simulink model "dynamic_mask_example"  (R2013a)
settings: Solver=VariableStepDiscrete  StartTime=0.0  StopTime=10.0  RelTol=1e-3
settings Model: Creator=bbhattac  LastModifiedBy=bbhattac

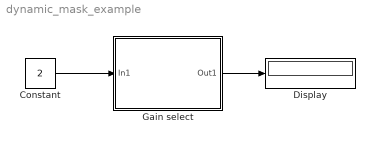
== system dynamic_mask_example ==
  Constant : Constant  Value=2
  Display : Display
  Gain select : Subsystem  mask{gain=2, val=2}
      mask prompts: val "Value:"
      mask TypeOptions gain: 2 | 5 | User-defined
      mask Callback gain:
      | maskStr = get_param(gcb,'MaskValues');
      | if strcmp(maskStr{1}(1),'U'),
      |     set_param(gcb,'MaskVisibilities',{'on';'on'}),
      | else
      |     set_param(gcb,'MaskVisibilities',{'on';'off'}),
      | 
      |     maskStr{2}=maskStr{1};
      |     set_param(gcb,'MaskValues',maskStr);
      | end
  wires:
  Gain select/1(Out1) -> Display/1
  Constant/1 -> Gain select/1(In1)

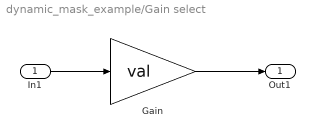
== system dynamic_mask_example/Gain select ==
  In1 : Inport
  Gain : Gain  Gain=val
  Out1 : Outport
  wires:
  Gain/1 -> Out1/1
  In1/1 -> Gain/1
